simulink library "uavsimBlockset_Zagi_Aerandpropulsion"  (Simulink 8.4)
settings: Solver=ode45  StartTime=0.0  StopTime=10.0  RelTol=1e-3
undefined symbols (not defined in the file): uavsim
libraries: uavsimBlockset_LinearAerodynamicCoefficient x6, uavsimBlockset_LiftCoefficientWithStall x1, aerolibadyn x1, uavsimBlockset_DerivedAerodynamicConditions x1
settings Model: Creator=mstolle  LastModifiedBy=j.bolting

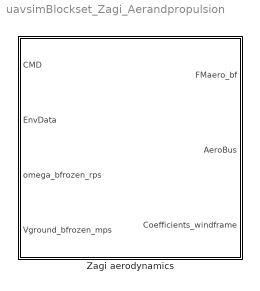
== system uavsimBlockset_Zagi_Aerandpropulsion ==
  Zagi aerodynamics : Subsystem

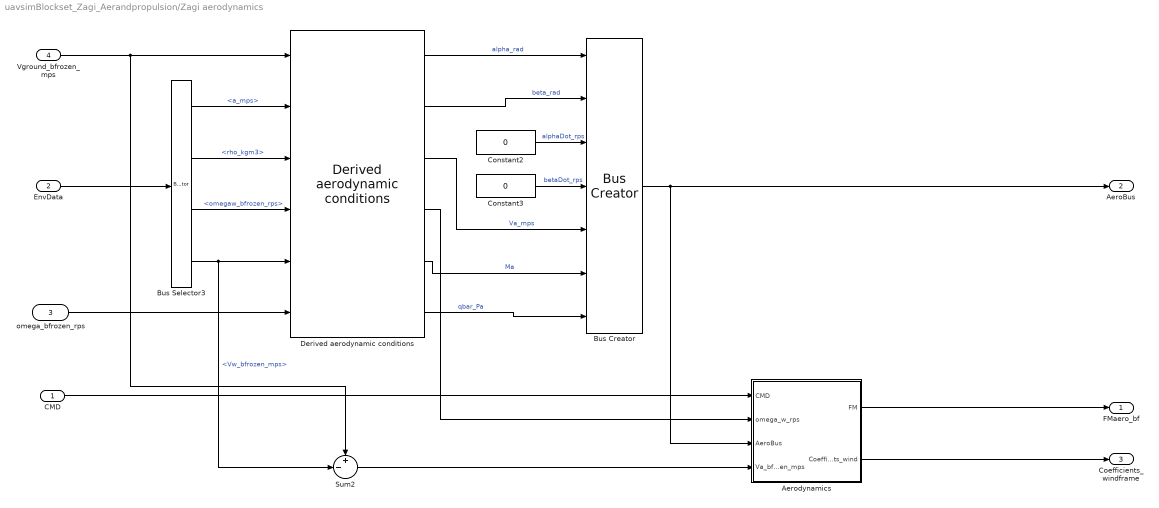
== system uavsimBlockset_Zagi_Aerandpropulsion/Zagi aerodynamics ==
  CMD : Inport  OutDataTypeStr=Bus: CMD
  EnvData : Inport  Port=2  OutDataTypeStr=Bus: Environment
  omega_bfrozen_rps : Inport  Port=3
  Vground_bfrozen_mps : Inport  Port=4
  Aerodynamics : Subsystem
  Bus Selector3 : BusSelector  OutputSignals=a_mps,rho_kgm3,omegaw_bfrozen_rps,Vw_bfrozen_mps
  Bus Creator : BusCreator  Inputs=7
  Constant2 : Constant  Value=0
  Constant3 : Constant  Value=0
  Derived aerodynamic conditions : uavsimBlockset_DerivedAerodynamicConditions/Derived aerodynamic conditions
  Sum2 : Sum  Inputs=+-|  SaturateOnIntegerOverflow=on  InputSameDT=on  OutDataTypeStr=Inherit: Same as first input
  FMaero_bf : Outport
  AeroBus : Outport  Port=2  OutDataTypeStr=Bus: Aero
  Coefficients_windframe : Outport  Port=3
  wires:
  EnvData/1 -> Bus Selector3/1
  omega_bfrozen_rps/1 -> Derived aerodynamic conditions/6
  Aerodynamics/1(FM) -> FMaero_bf/1
  CMD/1 -> Aerodynamics/1(CMD)
  Aerodynamics/2(Coefficients_wind) -> Coefficients_windframe/1
  Bus Selector3/1 -> Derived aerodynamic conditions/2  "<a_mps>"
  Bus Selector3/2 -> Derived aerodynamic conditions/3  "<rho_kgm3>"
  Bus Selector3/3 -> Derived aerodynamic conditions/4  "<omegaw_bfrozen_rps>"
  Bus Selector3/4 -> Derived aerodynamic conditions/5, Sum2/2  "<Vw_bfrozen_mps>"
  Constant2/1 -> Bus Creator/3  "alphaDot_rps"
  Constant3/1 -> Bus Creator/4  "betaDot_rps"
  Vground_bfrozen_mps/1 -> Sum2/1, Derived aerodynamic conditions/1
  Derived aerodynamic conditions/1 -> Bus Creator/1  "alpha_rad"
  Derived aerodynamic conditions/2 -> Bus Creator/2  "beta_rad"
  Derived aerodynamic conditions/3 -> Bus Creator/5  "Va_mps"
  Derived aerodynamic conditions/5 -> Bus Creator/6  "Ma"
  Derived aerodynamic conditions/6 -> Bus Creator/7  "qbar_Pa"
  Bus Creator/1 -> AeroBus/1, Aerodynamics/3(AeroBus)
  Derived aerodynamic conditions/4 -> Aerodynamics/2(omega_w_rps)
  Sum2/1 -> Aerodynamics/4(Va_bfrozen_mps)

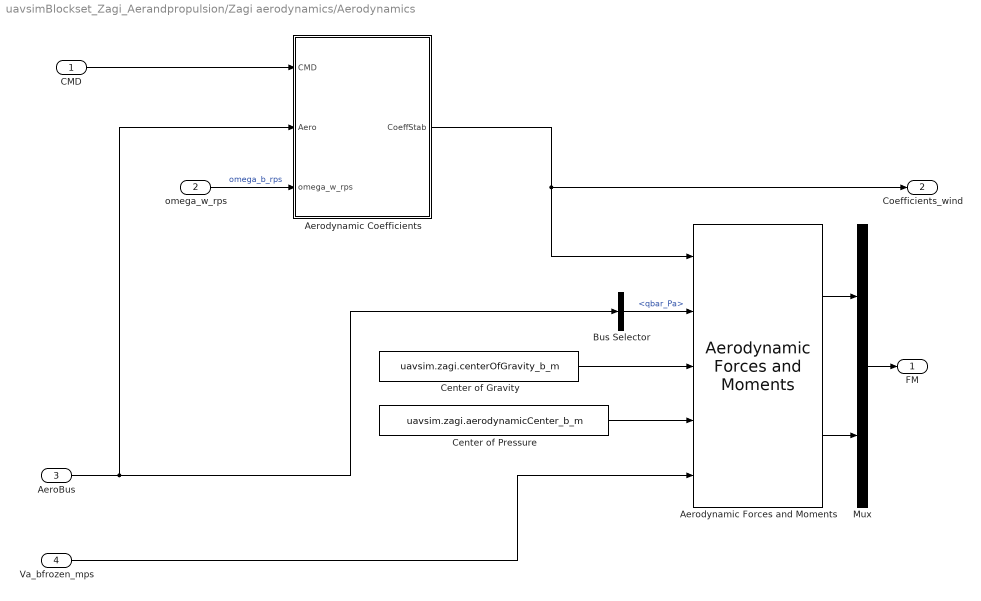
== system uavsimBlockset_Zagi_Aerandpropulsion/Zagi aerodynamics/Aerodynamics ==
  CMD : Inport  OutDataTypeStr=Bus: CMD
  omega_w_rps : Inport  Port=2
  AeroBus : Inport  Port=3  OutDataTypeStr=Bus: Aero
  Va_bfrozen_mps : Inport  Port=4
  Aerodynamic Coefficients : Subsystem
  "Aerodynamic Forces and Moments " : aerolibadyn/Aerodynamic Forces and Moments   inputAxes=Wind  outputForceAxes=Body  outputMomentAxes=Body  S=uavsim.zagi.S  b=uavsim.zagi.b  cbar=uavsim.zagi.c
  Bus Selector : BusSelector  OutputSignals=qbar_Pa
  Center of Gravity : Constant  Value=uavsim.zagi.centerOfGravity_b_m  SampleTime=0
  Center of Pressure : Constant  Value=uavsim.zagi.aerodynamicCenter_b_m  SampleTime=0
  Mux : Mux  Inputs=2
  FM : Outport
  Coefficients_wind : Outport  Port=2
  wires:
  AeroBus/1 -> Aerodynamic Coefficients/2(Aero), Bus Selector/1
  "Aerodynamic Forces and Moments "/2 -> Mux/2
  "Aerodynamic Forces and Moments "/1 -> Mux/1
  Center of Gravity/1 -> "Aerodynamic Forces and Moments "/3
  Center of Pressure/1 -> "Aerodynamic Forces and Moments "/4
  Aerodynamic Coefficients/1(CoeffStab) -> Coefficients_wind/1, "Aerodynamic Forces and Moments "/1
  CMD/1 -> Aerodynamic Coefficients/1(CMD)
  Mux/1 -> FM/1
  Bus Selector/1 -> "Aerodynamic Forces and Moments "/2  "<qbar_Pa>"
  omega_w_rps/1 -> Aerodynamic Coefficients/3(omega_w_rps)  "omega_b_rps"
  Va_bfrozen_mps/1 -> "Aerodynamic Forces and Moments "/5

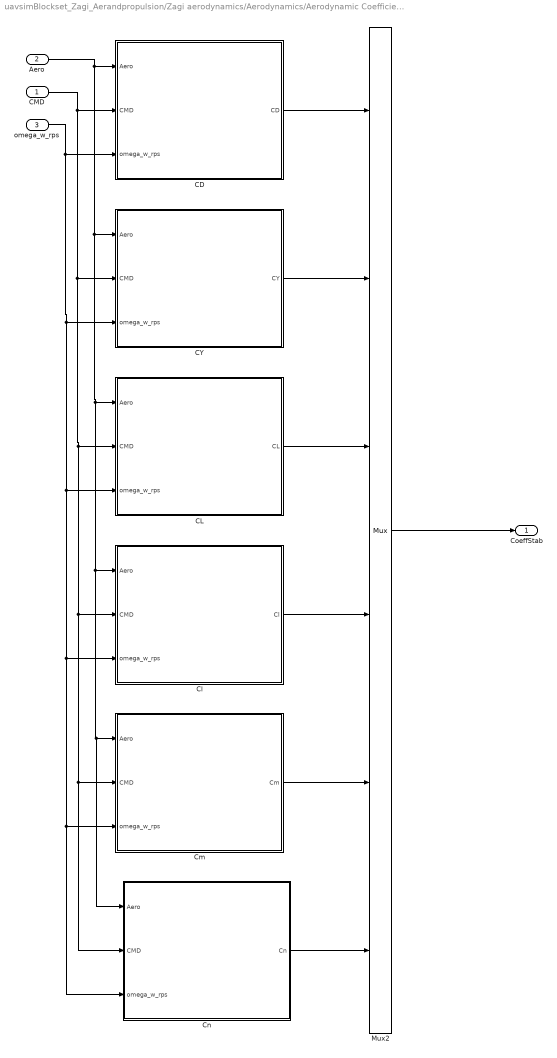
== system uavsimBlockset_Zagi_Aerandpropulsion/Zagi aerodynamics/Aerodynamics/Aerodynamic Coefficients ==
  CMD : Inport
  Aero : Inport  Port=2  OutDataTypeStr=Bus: Aero
  omega_w_rps : Inport  Port=3
  CD : Subsystem
  CL : Subsystem
  CY : Subsystem
  Cl : Subsystem
  Cm : Subsystem
  Cn : Subsystem
  Mux2 : Mux  Inputs=6
  CoeffStab : Outport
  wires:
  Mux2/1 -> CoeffStab/1
  omega_w_rps/1 -> Cn/3(omega_w_rps), Cm/3(omega_w_rps), Cl/3(omega_w_rps), CL/3(omega_w_rps), CY/3(omega_w_rps), CD/3(omega_w_rps)
  CMD/1 -> Cn/2(CMD), Cm/2(CMD), Cl/2(CMD), CL/2(CMD), CY/2(CMD), CD/2(CMD)
  Aero/1 -> Cn/1(Aero), Cm/1(Aero), Cl/1(Aero), CL/1(Aero), CY/1(Aero), CD/1(Aero)
  CL/1(CL) -> Mux2/3
  CD/1(CD) -> Mux2/1
  Cm/1(Cm) -> Mux2/5
  Cn/1(Cn) -> Mux2/6
  Cl/1(Cl) -> Mux2/4
  CY/1(CY) -> Mux2/2

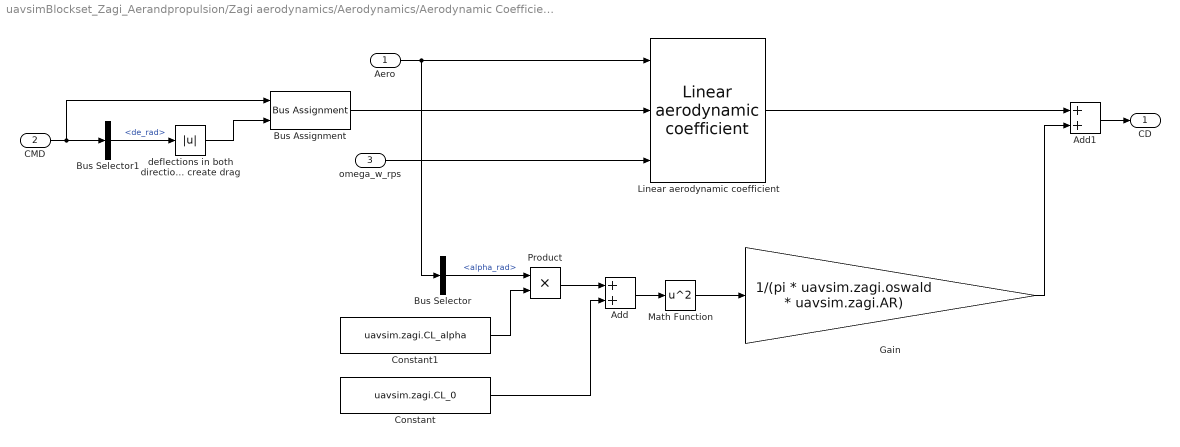
== system uavsimBlockset_Zagi_Aerandpropulsion/Zagi aerodynamics/Aerodynamics/Aerodynamic Coefficients/CD ==
  Aero : Inport  OutDataTypeStr=Bus: Aero
  CMD : Inport  Port=2  OutDataTypeStr=Bus: CMD
  omega_w_rps : Inport  Port=3
  Add : Sum
  Add1 : Sum
  Bus Assignment : BusAssignment  AssignedSignals=de_rad
  Bus Selector : BusSelector  OutputSignals=alpha_rad
  Bus Selector1 : BusSelector  OutputSignals=de_rad
  Constant : Constant  Value=uavsim.zagi.CL_0
  Constant1 : Constant  Value=uavsim.zagi.CL_alpha
  Gain : Gain  Gain=1/(pi * uavsim.zagi.oswald * uavsim.zagi.AR)
  Linear aerodynamic coefficient : uavsimBlockset_LinearAerodynamicCoefficient/Linear aerodynamic coefficient  mask_C_0=uavsim.zagi.CD_0  mask_C_alpha=0  mask_C_beta=0  mask_C_alphaDot=0  mask_C_betaDot=0  mask_C_p=0  mask_C_q=0  mask_C_r=0  mask_C_delta_a=0  mask_C_delta_e=uavsim.zagi.CD_de  mask_C_delta_r=0  mask_C_delta_f=0  mask_C_Mach=0
  Math Function : Math  Operator=square  SaturateOnIntegerOverflow=on
  Product : Product  RndMeth=Zero
  deflections in both directions always create drag : Abs
  CD : Outport
  wires:
  Constant/1 -> Add/2
  Add/1 -> Math Function/1
  Math Function/1 -> Gain/1
  Linear aerodynamic coefficient/1 -> Add1/1
  Add1/1 -> CD/1
  Gain/1 -> Add1/2
  Aero/1 -> Bus Selector/1, Linear aerodynamic coefficient/1
  omega_w_rps/1 -> Linear aerodynamic coefficient/3
  Bus Selector/1 -> Product/1  "<alpha_rad>"
  Product/1 -> Add/1
  Constant1/1 -> Product/2
  CMD/1 -> Bus Assignment/1, Bus Selector1/1
  Bus Selector1/1 -> deflections in both directions always create drag/1  "<de_rad>"
  deflections in both directions always create drag/1 -> Bus Assignment/2
  Bus Assignment/1 -> Linear aerodynamic coefficient/2

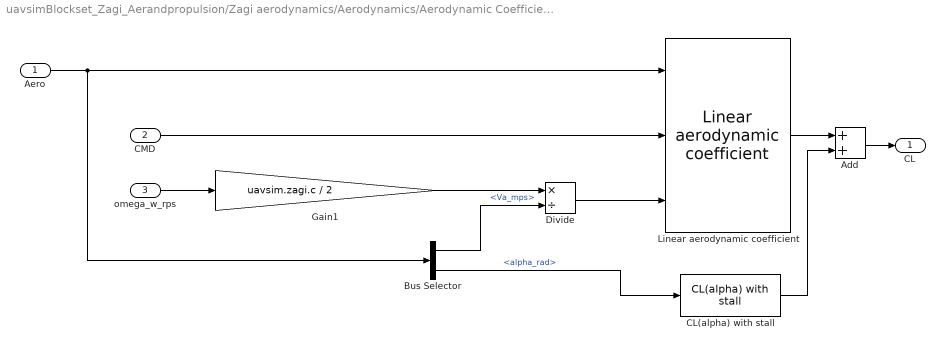
== system uavsimBlockset_Zagi_Aerandpropulsion/Zagi aerodynamics/Aerodynamics/Aerodynamic Coefficients/CL ==
  Aero : Inport  OutDataTypeStr=Bus: Aero
  CMD : Inport  Port=2  OutDataTypeStr=Bus: CMD
  omega_w_rps : Inport  Port=3
  Add : Sum
  Bus Selector : BusSelector  OutputSignals=Va_mps,alpha_rad
  CL(alpha) with stall : uavsimBlockset_LiftCoefficientWithStall/CL(alpha) with stall  mask_M=uavsim.zagi.stall.M  mask_alpha0=uavsim.zagi.alpha0  mask_CL_0=uavsim.zagi.CL_0  mask_CL_alpha=uavsim.zagi.CL_alpha
  Divide : Product  Inputs=*/
  Gain1 : Gain  Gain=uavsim.zagi.c / 2
  Linear aerodynamic coefficient : uavsimBlockset_LinearAerodynamicCoefficient/Linear aerodynamic coefficient  mask_C_0=0  mask_C_alpha=0  mask_C_beta=0  mask_C_alphaDot=0  mask_C_betaDot=0  mask_C_p=0  mask_C_q=uavsim.zagi.CL_q  mask_C_r=0  mask_C_delta_a=0  mask_C_delta_e=uavsim.zagi.CL_de  mask_C_delta_r=0  mask_C_delta_f=0  mask_C_Mach=0
  CL : Outport
  wires:
  Linear aerodynamic coefficient/1 -> Add/1
  Divide/1 -> Linear aerodynamic coefficient/3
  Bus Selector/1 -> Divide/2  "<Va_mps>"
  Gain1/1 -> Divide/1
  CMD/1 -> Linear aerodynamic coefficient/2
  omega_w_rps/1 -> Gain1/1
  Aero/1 -> Linear aerodynamic coefficient/1, Bus Selector/1
  Bus Selector/2 -> CL(alpha) with stall/1  "<alpha_rad>"
  CL(alpha) with stall/1 -> Add/2
  Add/1 -> CL/1

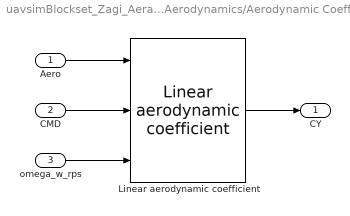
== system uavsimBlockset_Zagi_Aerandpropulsion/Zagi aerodynamics/Aerodynamics/Aerodynamic Coefficients/CY ==
  Aero : Inport  OutDataTypeStr=Bus: Aero
  CMD : Inport  Port=2  OutDataTypeStr=Bus: CMD
  omega_w_rps : Inport  Port=3
  Linear aerodynamic coefficient : uavsimBlockset_LinearAerodynamicCoefficient/Linear aerodynamic coefficient  mask_C_0=0  mask_C_alpha=0  mask_C_beta=uavsim.zagi.CY_beta  mask_C_alphaDot=0  mask_C_betaDot=0  mask_C_p=0  mask_C_q=0  mask_C_r=0  mask_C_delta_a=0  mask_C_delta_e=0  mask_C_delta_r=0  mask_C_delta_f=0  mask_C_Mach=0
  CY : Outport
  wires:
  CMD/1 -> Linear aerodynamic coefficient/2
  Aero/1 -> Linear aerodynamic coefficient/1
  Linear aerodynamic coefficient/1 -> CY/1
  omega_w_rps/1 -> Linear aerodynamic coefficient/3

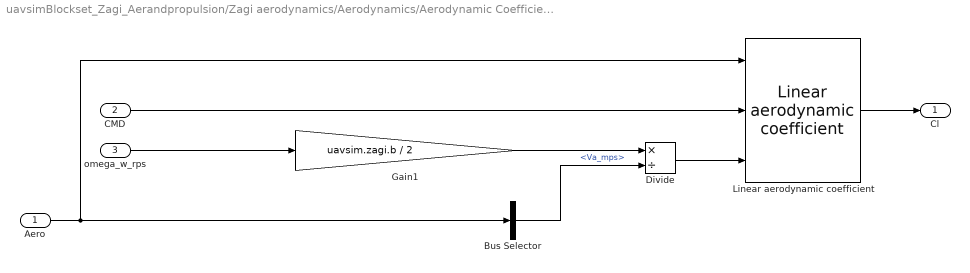
== system uavsimBlockset_Zagi_Aerandpropulsion/Zagi aerodynamics/Aerodynamics/Aerodynamic Coefficients/Cl ==
  Aero : Inport  OutDataTypeStr=Bus: Aero
  CMD : Inport  Port=2  OutDataTypeStr=Bus: CMD
  omega_w_rps : Inport  Port=3
  Bus Selector : BusSelector  OutputSignals=Va_mps
  Divide : Product  Inputs=*/
  Gain1 : Gain  Gain=uavsim.zagi.b / 2
  Linear aerodynamic coefficient : uavsimBlockset_LinearAerodynamicCoefficient/Linear aerodynamic coefficient  mask_C_0=0  mask_C_alpha=0  mask_C_beta=uavsim.zagi.Cl_beta  mask_C_alphaDot=0  mask_C_betaDot=0  mask_C_p=uavsim.zagi.Cl_p  mask_C_q=0  mask_C_r=uavsim.zagi.Cl_r  mask_C_delta_a=uavsim.zagi.Cl_da  mask_C_delta_e=0  mask_C_delta_r=0  mask_C_delta_f=0  mask_C_Mach=0
  Cl : Outport
  wires:
  Aero/1 -> Bus Selector/1, Linear aerodynamic coefficient/1
  omega_w_rps/1 -> Gain1/1
  CMD/1 -> Linear aerodynamic coefficient/2
  Gain1/1 -> Divide/1
  Bus Selector/1 -> Divide/2  "<Va_mps>"
  Divide/1 -> Linear aerodynamic coefficient/3
  Linear aerodynamic coefficient/1 -> Cl/1

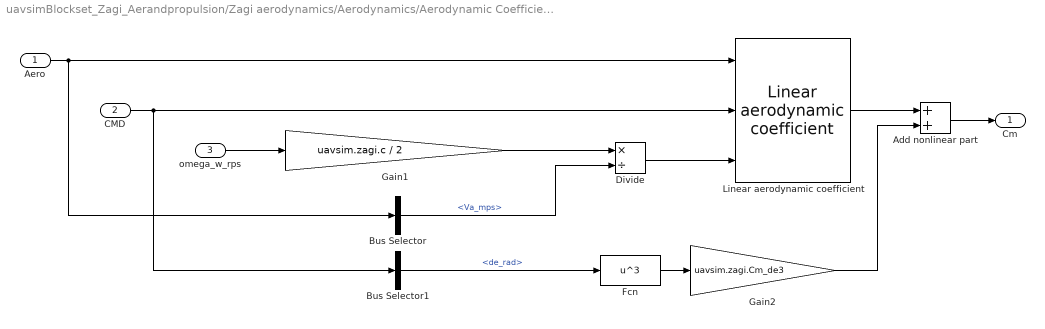
== system uavsimBlockset_Zagi_Aerandpropulsion/Zagi aerodynamics/Aerodynamics/Aerodynamic Coefficients/Cm ==
  Aero : Inport  OutDataTypeStr=Bus: Aero
  CMD : Inport  Port=2  OutDataTypeStr=Bus: CMD
  omega_w_rps : Inport  Port=3
  Add nonlinear part : Sum
  Bus Selector : BusSelector  OutputSignals=Va_mps
  Bus Selector1 : BusSelector  OutputSignals=de_rad
  Divide : Product  Inputs=*/
  Fcn : Fcn  Expr=u^3
  Gain1 : Gain  Gain=uavsim.zagi.c / 2
  Gain2 : Gain  Gain=uavsim.zagi.Cm_de3
  Linear aerodynamic coefficient : uavsimBlockset_LinearAerodynamicCoefficient/Linear aerodynamic coefficient  mask_C_0=uavsim.zagi.Cm_0  mask_C_alpha=uavsim.zagi.Cm_alpha  mask_C_beta=0  mask_C_alphaDot=0  mask_C_betaDot=0  mask_C_p=0  mask_C_q=uavsim.zagi.Cm_q  mask_C_r=0  mask_C_delta_a=0  mask_C_delta_e=uavsim.zagi.Cm_de  mask_C_delta_r=0  mask_C_delta_f=0  mask_C_Mach=0
  Cm : Outport
  wires:
  Aero/1 -> Linear aerodynamic coefficient/1, Bus Selector/1
  omega_w_rps/1 -> Gain1/1
  CMD/1 -> Linear aerodynamic coefficient/2, Bus Selector1/1
  Gain1/1 -> Divide/1
  Bus Selector/1 -> Divide/2  "<Va_mps>"
  Divide/1 -> Linear aerodynamic coefficient/3
  Linear aerodynamic coefficient/1 -> Add nonlinear part/1
  Add nonlinear part/1 -> Cm/1
  Fcn/1 -> Gain2/1
  Gain2/1 -> Add nonlinear part/2
  Bus Selector1/1 -> Fcn/1  "<de_rad>"

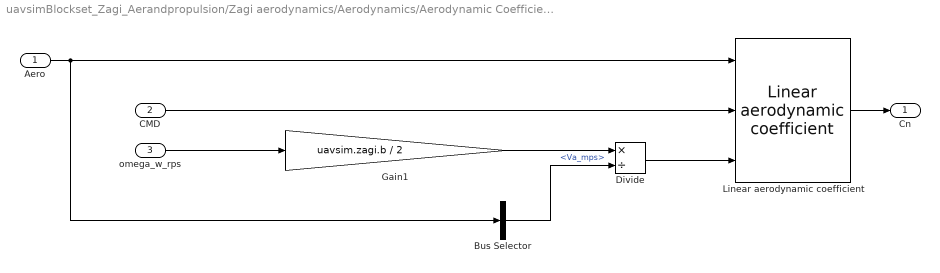
== system uavsimBlockset_Zagi_Aerandpropulsion/Zagi aerodynamics/Aerodynamics/Aerodynamic Coefficients/Cn ==
  Aero : Inport  OutDataTypeStr=Bus: Aero
  CMD : Inport  Port=2  OutDataTypeStr=Bus: CMD
  omega_w_rps : Inport  Port=3
  Bus Selector : BusSelector  OutputSignals=Va_mps
  Divide : Product  Inputs=*/
  Gain1 : Gain  Gain=uavsim.zagi.b / 2
  Linear aerodynamic coefficient : uavsimBlockset_LinearAerodynamicCoefficient/Linear aerodynamic coefficient  mask_C_0=0  mask_C_alpha=0  mask_C_beta=uavsim.zagi.Cn_beta  mask_C_alphaDot=0  mask_C_betaDot=0  mask_C_p=uavsim.zagi.Cn_p  mask_C_q=0  mask_C_r=uavsim.zagi.Cn_r  mask_C_delta_a=uavsim.zagi.Cn_da  mask_C_delta_e=0  mask_C_delta_r=0  mask_C_delta_f=0  mask_C_Mach=0
  Cn : Outport
  wires:
  Linear aerodynamic coefficient/1 -> Cn/1
  Divide/1 -> Linear aerodynamic coefficient/3
  Bus Selector/1 -> Divide/2  "<Va_mps>"
  Gain1/1 -> Divide/1
  CMD/1 -> Linear aerodynamic coefficient/2
  omega_w_rps/1 -> Gain1/1
  Aero/1 -> Bus Selector/1, Linear aerodynamic coefficient/1
